simulink model "roach2_fengine_nlb"  (R2013b)
settings: Solver=VariableStepDiscrete  SolverMode=SingleTasking  StartTime=0.0  StopTime=10.0  RelTol=1e-3
undefined symbols (not defined in the file or in its folder): sfp
libraries: xbsIndex_r4 x3316, xps_library x74, casper_library_sources x16, casper_library_misc x7
(part 4 of 38)

== system roach2_fengine_nlb/eq/7 ==
  note: Counter has length nchan=number of channels of the fft.
      | BRAM has length nchan as well. Every input/channel
      | has its own eq value.
      | Top half of the BRAM, has coefficients for first input,
      | second half for the rest.
  note: shared brams have a latency of three
  in : Inport
  sync : Inport  Port=2
  Constant4 : xbsIndex_r4/Constant  const=0  gui_display_data_type=Fixed-point  arith_type=Unsigned  n_bits=18  bin_pt=0  preci_type=Single  exp_width=8  frac_width=24  explicit_period=on  period=1  equ=P=C  opselect=C  inp2=PCIN>>17  opr=+  inp1=P  carry=CIN  dbl_ovrd=off  block_type=constant
  Constant5 : xbsIndex_r4/Constant  const=0  gui_display_data_type=Fixed-point  arith_type=Boolean  n_bits=1  bin_pt=0  preci_type=Single  exp_width=8  frac_width=24  explicit_period=on  period=1  equ=P=C  opselect=C  inp2=PCIN>>17  opr=+  inp1=P  carry=CIN  dbl_ovrd=off  block_type=constant
  Counter : xbsIndex_r4/Counter  cnt_type=Free Running  cnt_to=Inf  operation=Up  start_count=0  cnt_by_val=1  arith_type=Unsigned  n_bits=nchan  bin_pt=0  load_pin=off  rst=on  en=off  explicit_period=off  period=1  dbl_ovrd=off  use_behavioral_HDL=off  implementation=Fabric  use_rpm=on  block_type=counter
      settings: xl_area=[0, 0, 0, 0, 0, 0, 0]
  Delay1 : xbsIndex_r4/Delay  rst=off  infoeditControl=Selection of Reset will increase slice count due to use of real FFs and instead of SRLs  en=off  latency=4  dbl_ovrd=off  reg_retiming=on  block_type=delay
      settings: xl_area=[0, 0, 0, 0, 0, 0, 0]
  Delay11 : xbsIndex_r4/Delay  rst=off  infoeditControl=Selection of Reset will increase slice count due to use of real FFs and instead of SRLs  en=off  latency=4  dbl_ovrd=off  reg_retiming=on  block_type=delay
      settings: xl_area=[0, 0, 0, 0, 0, 0, 0]
  Delay2 : xbsIndex_r4/Delay  rst=off  infoeditControl=Selection of Reset will increase slice count due to use of real FFs and instead of SRLs  en=off  latency=3  dbl_ovrd=off  reg_retiming=off  block_type=delay
      settings: xl_area=[0, 0, 0, 0, 0, 0, 0]
  Delay3 : xbsIndex_r4/Delay  rst=off  infoeditControl=Selection of Reset will increase slice count due to use of real FFs and instead of SRLs  en=off  latency=4  dbl_ovrd=off  reg_retiming=on  block_type=delay
      settings: xl_area=[0, 0, 0, 0, 0, 0, 0]
  Delay4 : xbsIndex_r4/Delay  rst=off  infoeditControl=Selection of Reset will increase slice count due to use of real FFs and instead of SRLs  en=off  latency=5  dbl_ovrd=off  reg_retiming=off  block_type=delay
      settings: xl_area=[0, 0, 0, 0, 0, 0, 0]
  Delay5 : xbsIndex_r4/Delay  rst=off  infoeditControl=Selection of Reset will increase slice count due to use of real FFs and instead of SRLs  en=off  latency=3  dbl_ovrd=off  reg_retiming=off  block_type=delay
      settings: xl_area=[0, 0, 0, 0, 0, 0, 0]
  Slice1 : xbsIndex_r4/Slice  nbits=18  boolean_output=off  mode=Lower Bit Location + Width  bit1=0  base1=MSB of Input  bit0=0  base0=LSB of Input  dbl_ovrd=off  block_type=slice
      settings: block_version=10.1.3
  coeffs : Subsystem  Tag=xps:bram  AncestorBlock=xps_library/Shared BRAM  mask{arith_type=Unsigned, addr_width=nchan, data_width=32, reg_prim_output=on, reg_core_output=on, optimization=Minimum_Area, data_bin_pt=0, init_vals=[0:2^10-1], sample_rate=1}
      mask prompts: arith_type "Output Data Type"; addr_width "Address width"; data_width "Data Width"; reg_prim_output "Register Primitive Output"; reg_core_output "Register Core Output"; data_bin_pt "Data Binary Point"; init_vals "Initial 32-bit values (simulation only)"; sample_rate "Sample rate"
      mask init:
      | shared_bram_mask;
      mask TypeOptions arith_type: Unsigned | Signed  (2's comp)
      mask TypeOptions data_width: 8 | 16 | 32 | 64 | 128
      mask TypeOptions optimization: Minimum_Area | Low_Power
  round : Subsystem
      settings: AttributesFormatString=latency=5
  dout : Outport
  sync_out : Outport  Port=2
  clip : Outport  Port=3
  wires:
  Constant4/1 -> coeffs/2(data_in)
  Constant5/1 -> coeffs/3(we)
  sync/1 -> Counter/1, Delay5/1
  round/1(dout) -> dout/1
  in/1 -> Delay2/1
  Delay4/1 -> sync_out/1
  round/2(clip) -> clip/1
  coeffs/1(data_out) -> Slice1/1
  Counter/1 -> coeffs/1(addr)
  Delay1/1 -> round/2(scale)
  Slice1/1 -> Delay1/1
  Delay11/1 -> round/1(din)
  Delay2/1 -> Delay11/1
  Delay3/1 -> Delay4/1
  Delay5/1 -> Delay3/1

== system roach2_fengine_nlb/eq/8 ==
  note: shared brams have a latency of three
  note: Counter has length nchan=number of channels of the fft.
      | BRAM has length nchan as well. Every input/channel
      | has its own eq value.
      | Top half of the BRAM, has coefficients for first input,
      | second half for the rest.
  in : Inport
  sync : Inport  Port=2
  Constant4 : xbsIndex_r4/Constant  const=0  gui_display_data_type=Fixed-point  arith_type=Unsigned  n_bits=18  bin_pt=0  preci_type=Single  exp_width=8  frac_width=24  explicit_period=on  period=1  equ=P=C  opselect=C  inp2=PCIN>>17  opr=+  inp1=P  carry=CIN  dbl_ovrd=off  block_type=constant
  Constant5 : xbsIndex_r4/Constant  const=0  gui_display_data_type=Fixed-point  arith_type=Boolean  n_bits=1  bin_pt=0  preci_type=Single  exp_width=8  frac_width=24  explicit_period=on  period=1  equ=P=C  opselect=C  inp2=PCIN>>17  opr=+  inp1=P  carry=CIN  dbl_ovrd=off  block_type=constant
  Counter : xbsIndex_r4/Counter  cnt_type=Free Running  cnt_to=Inf  operation=Up  start_count=0  cnt_by_val=1  arith_type=Unsigned  n_bits=nchan  bin_pt=0  load_pin=off  rst=on  en=off  explicit_period=off  period=1  dbl_ovrd=off  use_behavioral_HDL=off  implementation=Fabric  use_rpm=on  block_type=counter
      settings: xl_area=[0, 0, 0, 0, 0, 0, 0]
  Delay1 : xbsIndex_r4/Delay  rst=off  infoeditControl=Selection of Reset will increase slice count due to use of real FFs and instead of SRLs  en=off  latency=4  dbl_ovrd=off  reg_retiming=on  block_type=delay
      settings: xl_area=[0, 0, 0, 0, 0, 0, 0]
  Delay11 : xbsIndex_r4/Delay  rst=off  infoeditControl=Selection of Reset will increase slice count due to use of real FFs and instead of SRLs  en=off  latency=4  dbl_ovrd=off  reg_retiming=on  block_type=delay
      settings: xl_area=[0, 0, 0, 0, 0, 0, 0]
  Delay2 : xbsIndex_r4/Delay  rst=off  infoeditControl=Selection of Reset will increase slice count due to use of real FFs and instead of SRLs  en=off  latency=3  dbl_ovrd=off  reg_retiming=off  block_type=delay
      settings: xl_area=[0, 0, 0, 0, 0, 0, 0]
  Delay3 : xbsIndex_r4/Delay  rst=off  infoeditControl=Selection of Reset will increase slice count due to use of real FFs and instead of SRLs  en=off  latency=4  dbl_ovrd=off  reg_retiming=on  block_type=delay
      settings: xl_area=[0, 0, 0, 0, 0, 0, 0]
  Delay4 : xbsIndex_r4/Delay  rst=off  infoeditControl=Selection of Reset will increase slice count due to use of real FFs and instead of SRLs  en=off  latency=5  dbl_ovrd=off  reg_retiming=off  block_type=delay
      settings: xl_area=[0, 0, 0, 0, 0, 0, 0]
  Delay5 : xbsIndex_r4/Delay  rst=off  infoeditControl=Selection of Reset will increase slice count due to use of real FFs and instead of SRLs  en=off  latency=3  dbl_ovrd=off  reg_retiming=off  block_type=delay
      settings: xl_area=[0, 0, 0, 0, 0, 0, 0]
  Slice1 : xbsIndex_r4/Slice  nbits=18  boolean_output=off  mode=Lower Bit Location + Width  bit1=0  base1=MSB of Input  bit0=0  base0=LSB of Input  dbl_ovrd=off  block_type=slice
      settings: block_version=10.1.3
  coeffs : Subsystem  Tag=xps:bram  AncestorBlock=xps_library/Shared BRAM  mask{arith_type=Unsigned, addr_width=nchan, data_width=32, reg_prim_output=on, reg_core_output=on, optimization=Minimum_Area, data_bin_pt=0, init_vals=[0:2^10-1], sample_rate=1}
      mask prompts: arith_type "Output Data Type"; addr_width "Address width"; data_width "Data Width"; reg_prim_output "Register Primitive Output"; reg_core_output "Register Core Output"; data_bin_pt "Data Binary Point"; init_vals "Initial 32-bit values (simulation only)"; sample_rate "Sample rate"
      mask init:
      | shared_bram_mask;
      mask TypeOptions arith_type: Unsigned | Signed  (2's comp)
      mask TypeOptions data_width: 8 | 16 | 32 | 64 | 128
      mask TypeOptions optimization: Minimum_Area | Low_Power
  round : Subsystem
      settings: AttributesFormatString=latency=5
  dout : Outport
  sync_out : Outport  Port=2
  clip : Outport  Port=3
  wires:
  Delay5/1 -> Delay3/1
  Delay3/1 -> Delay4/1
  Delay2/1 -> Delay11/1
  Delay11/1 -> round/1(din)
  Slice1/1 -> Delay1/1
  Delay1/1 -> round/2(scale)
  Counter/1 -> coeffs/1(addr)
  coeffs/1(data_out) -> Slice1/1
  round/2(clip) -> clip/1
  Delay4/1 -> sync_out/1
  in/1 -> Delay2/1
  round/1(dout) -> dout/1
  sync/1 -> Delay5/1, Counter/1
  Constant5/1 -> coeffs/3(we)
  Constant4/1 -> coeffs/2(data_in)

== system roach2_fengine_nlb/eq/9 ==
  note: shared brams have a latency of three
  note: Counter has length nchan=number of channels of the fft.
      | BRAM has length nchan as well. Every input/channel
      | has its own eq value.
      | Top half of the BRAM, has coefficients for first input,
      | second half for the rest.
  in : Inport
  sync : Inport  Port=2
  Constant4 : xbsIndex_r4/Constant  const=0  gui_display_data_type=Fixed-point  arith_type=Unsigned  n_bits=18  bin_pt=0  preci_type=Single  exp_width=8  frac_width=24  explicit_period=on  period=1  equ=P=C  opselect=C  inp2=PCIN>>17  opr=+  inp1=P  carry=CIN  dbl_ovrd=off  block_type=constant
  Constant5 : xbsIndex_r4/Constant  const=0  gui_display_data_type=Fixed-point  arith_type=Boolean  n_bits=1  bin_pt=0  preci_type=Single  exp_width=8  frac_width=24  explicit_period=on  period=1  equ=P=C  opselect=C  inp2=PCIN>>17  opr=+  inp1=P  carry=CIN  dbl_ovrd=off  block_type=constant
  Counter : xbsIndex_r4/Counter  cnt_type=Free Running  cnt_to=Inf  operation=Up  start_count=0  cnt_by_val=1  arith_type=Unsigned  n_bits=nchan  bin_pt=0  load_pin=off  rst=on  en=off  explicit_period=off  period=1  dbl_ovrd=off  use_behavioral_HDL=off  implementation=Fabric  use_rpm=on  block_type=counter
      settings: xl_area=[0, 0, 0, 0, 0, 0, 0]
  Delay1 : xbsIndex_r4/Delay  rst=off  infoeditControl=Selection of Reset will increase slice count due to use of real FFs and instead of SRLs  en=off  latency=4  dbl_ovrd=off  reg_retiming=on  block_type=delay
      settings: xl_area=[0, 0, 0, 0, 0, 0, 0]
  Delay11 : xbsIndex_r4/Delay  rst=off  infoeditControl=Selection of Reset will increase slice count due to use of real FFs and instead of SRLs  en=off  latency=4  dbl_ovrd=off  reg_retiming=on  block_type=delay
      settings: xl_area=[0, 0, 0, 0, 0, 0, 0]
  Delay2 : xbsIndex_r4/Delay  rst=off  infoeditControl=Selection of Reset will increase slice count due to use of real FFs and instead of SRLs  en=off  latency=3  dbl_ovrd=off  reg_retiming=off  block_type=delay
      settings: xl_area=[0, 0, 0, 0, 0, 0, 0]
  Delay3 : xbsIndex_r4/Delay  rst=off  infoeditControl=Selection of Reset will increase slice count due to use of real FFs and instead of SRLs  en=off  latency=4  dbl_ovrd=off  reg_retiming=on  block_type=delay
      settings: xl_area=[0, 0, 0, 0, 0, 0, 0]
  Delay4 : xbsIndex_r4/Delay  rst=off  infoeditControl=Selection of Reset will increase slice count due to use of real FFs and instead of SRLs  en=off  latency=5  dbl_ovrd=off  reg_retiming=off  block_type=delay
      settings: xl_area=[0, 0, 0, 0, 0, 0, 0]
  Delay5 : xbsIndex_r4/Delay  rst=off  infoeditControl=Selection of Reset will increase slice count due to use of real FFs and instead of SRLs  en=off  latency=3  dbl_ovrd=off  reg_retiming=off  block_type=delay
      settings: xl_area=[0, 0, 0, 0, 0, 0, 0]
  Slice1 : xbsIndex_r4/Slice  nbits=18  boolean_output=off  mode=Lower Bit Location + Width  bit1=0  base1=MSB of Input  bit0=0  base0=LSB of Input  dbl_ovrd=off  block_type=slice
      settings: block_version=10.1.3
  coeffs : Subsystem  Tag=xps:bram  AncestorBlock=xps_library/Shared BRAM  mask{arith_type=Unsigned, addr_width=nchan, data_width=32, reg_prim_output=on, reg_core_output=on, optimization=Minimum_Area, data_bin_pt=0, init_vals=[0:2^10-1], sample_rate=1}
      mask prompts: arith_type "Output Data Type"; addr_width "Address width"; data_width "Data Width"; reg_prim_output "Register Primitive Output"; reg_core_output "Register Core Output"; data_bin_pt "Data Binary Point"; init_vals "Initial 32-bit values (simulation only)"; sample_rate "Sample rate"
      mask init:
      | shared_bram_mask;
      mask TypeOptions arith_type: Unsigned | Signed  (2's comp)
      mask TypeOptions data_width: 8 | 16 | 32 | 64 | 128
      mask TypeOptions optimization: Minimum_Area | Low_Power
  round : Subsystem
      settings: AttributesFormatString=latency=5
  dout : Outport
  sync_out : Outport  Port=2
  clip : Outport  Port=3
  wires:
  Delay5/1 -> Delay3/1
  Delay3/1 -> Delay4/1
  Delay2/1 -> Delay11/1
  Delay11/1 -> round/1(din)
  Slice1/1 -> Delay1/1
  Delay1/1 -> round/2(scale)
  Counter/1 -> coeffs/1(addr)
  coeffs/1(data_out) -> Slice1/1
  round/2(clip) -> clip/1
  Delay4/1 -> sync_out/1
  in/1 -> Delay2/1
  round/1(dout) -> dout/1
  sync/1 -> Delay5/1, Counter/1
  Constant5/1 -> coeffs/3(we)
  Constant4/1 -> coeffs/2(data_in)

== system roach2_fengine_nlb/eq/eq_snap ==
  In1 : Inport
  In2 : Inport  Port=2
  In3 : Inport  Port=3
  In4 : Inport  Port=4
  BitBasher : xbsIndex_r4/BitBasher  bitexpr=|  display_expr=off  sr_1=1  arith_type1=Unsigned  bin_pt1=0  sr_2=2  arith_type2=Unsigned  bin_pt2=0  sr_3=3  arith_type3=Unsigned  bin_pt3=0  sr_4=4  arith_type4=Unsigned  bin_pt4=0  dbl_ovrd=off  block_type=bitbasher
      | <!DOCTYPE HTML PUBLIC "-//W3C//DTD HTML 4.0//EN" "http://www.w3.org/TR/REC-html40/strict.dtd">
      | <html><head><meta name="qrichtext" content="1" /><style type="text/css">
      | p, li { white-space: pre-wrap; }
      | </style></head><body style=" font-family:'Sans'; font-size:10pt; font-weight:400; font-style:normal;">
      | <p style=" margin-top:12px; margin-bottom:12px; margin-left:0px; margin-right:0px; -qt-block-indent:0; text-indent:0px;"><span style=" font-family:'MS Shell Dlg'; font-size:8pt;">w32={d8,c8,b8,a8}</span></p></body></html>
  Delay : xbsIndex_r4/Delay  rst=off  infoeditControl=Selection of Reset will increase slice count due to use of real FFs and instead of SRLs  en=off  latency=3  dbl_ovrd=off  reg_retiming=on  block_type=delay
  tag scope: eq_snap=global
  wires:
  BitBasher/1 -> Delay/1
  Delay/1 -> [eq_snap]
  In1/1 -> BitBasher/1
  In2/1 -> BitBasher/2
  In3/1 -> BitBasher/3
  In4/1 -> BitBasher/4

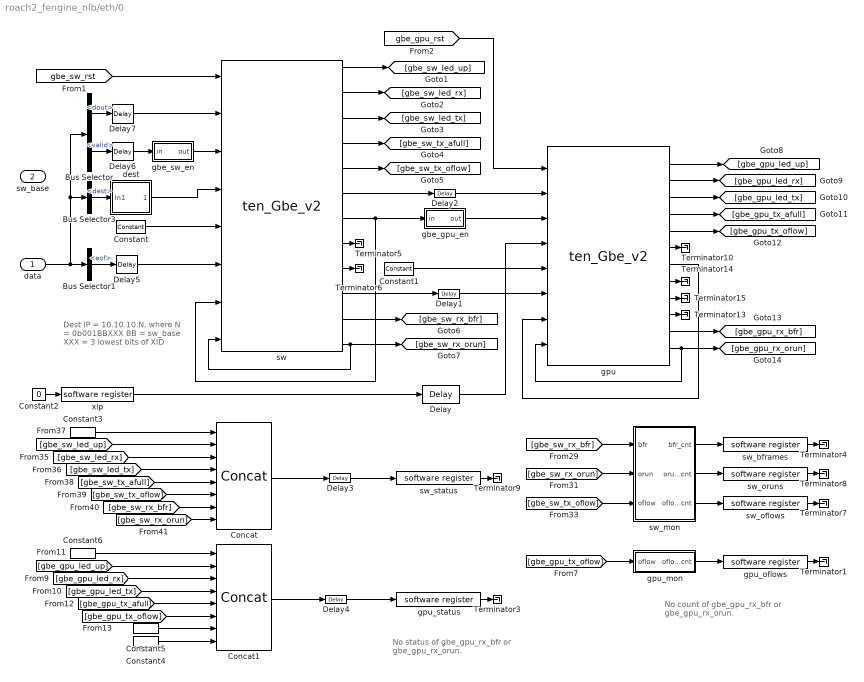
== system roach2_fengine_nlb/eth/0 ==
  note: Dest IP = 10.10.10.N, where
      | N = 0b001BBXXX
      | BB = sw_base
      | XXX = 3 lowest bits of XID
  note: No count of gbe_gpu_rx_bfr or gbe_gpu_rx_orun.
  note: No status of gbe_gpu_rx_bfr or gbe_gpu_rx_orun.
  data : Inport
  sw_base : Inport  Port=2
  Bus Selector : BusSelector  OutputSignals=dout,valid
  Bus Selector1 : BusSelector  OutputSignals=eof
  Bus Selector3 : BusSelector  OutputSignals=dest
  Concat : xbsIndex_r4/Concat  num_inputs=8  dbl_ovrd=off  block_type=concat
  Concat1 : xbsIndex_r4/Concat  num_inputs=8  dbl_ovrd=off  block_type=concat
  Constant : xbsIndex_r4/Constant  const=8511  gui_display_data_type=Fixed-point  arith_type=Unsigned  n_bits=16  bin_pt=0  preci_type=Single  exp_width=8  frac_width=24  explicit_period=on  period=1  equ=P=C  opselect=C  inp2=PCIN>>17  opr=+  inp1=P  carry=CIN  dbl_ovrd=off  block_type=constant
  Constant1 : xbsIndex_r4/Constant  const=8511  gui_display_data_type=Fixed-point  arith_type=Unsigned  n_bits=16  bin_pt=0  preci_type=Single  exp_width=8  frac_width=24  explicit_period=on  period=1  equ=P=C  opselect=C  inp2=PCIN>>17  opr=+  inp1=P  carry=CIN  dbl_ovrd=off  block_type=constant
  Constant2 : Constant  Value=0
  Constant3 : xbsIndex_r4/Constant  const=0  gui_display_data_type=Fixed-point  arith_type=Unsigned  n_bits=25  bin_pt=0  preci_type=Single  exp_width=8  frac_width=24  explicit_period=on  period=1  equ=P=C  opselect=C  inp2=PCIN>>17  opr=+  inp1=P  carry=CIN  dbl_ovrd=off  block_type=constant
      settings: block_version=11.4
  Constant4 : xbsIndex_r4/Constant  const=0  gui_display_data_type=Fixed-point  arith_type=Unsigned  n_bits=1  bin_pt=0  preci_type=Single  exp_width=8  frac_width=24  explicit_period=on  period=1  equ=P=C  opselect=C  inp2=PCIN>>17  opr=+  inp1=P  carry=CIN  dbl_ovrd=off  block_type=constant
      settings: block_version=11.4
  Constant5 : xbsIndex_r4/Constant  const=0  gui_display_data_type=Fixed-point  arith_type=Unsigned  n_bits=1  bin_pt=0  preci_type=Single  exp_width=8  frac_width=24  explicit_period=on  period=1  equ=P=C  opselect=C  inp2=PCIN>>17  opr=+  inp1=P  carry=CIN  dbl_ovrd=off  block_type=constant
      settings: block_version=11.4
  Constant6 : xbsIndex_r4/Constant  const=0  gui_display_data_type=Fixed-point  arith_type=Unsigned  n_bits=25  bin_pt=0  preci_type=Single  exp_width=8  frac_width=24  explicit_period=on  period=1  equ=P=C  opselect=C  inp2=PCIN>>17  opr=+  inp1=P  carry=CIN  dbl_ovrd=off  block_type=constant
      settings: block_version=11.4
  Delay{,1..4} (5 alike) : xbsIndex_r4/Delay  rst=off  infoeditControl=Selection of Reset will increase slice count due to use of real FFs and instead of SRLs  en=off  latency=1  dbl_ovrd=off  reg_retiming=off  block_type=delay
  Delay5 : xbsIndex_r4/Delay  rst=off  infoeditControl=Selection of Reset will increase slice count due to use of real FFs and instead of SRLs  en=off  latency=3  dbl_ovrd=off  reg_retiming=off  block_type=delay
  Delay6 : xbsIndex_r4/Delay  rst=off  infoeditControl=Selection of Reset will increase slice count due to use of real FFs and instead of SRLs  en=off  latency=3  dbl_ovrd=off  reg_retiming=off  block_type=delay
  Delay7 : xbsIndex_r4/Delay  rst=off  infoeditControl=Selection of Reset will increase slice count due to use of real FFs and instead of SRLs  en=off  latency=3  dbl_ovrd=off  reg_retiming=off  block_type=delay
  Terminator{1,3..10,13..15} (12 alike) : Terminator
  dest : Subsystem
  gbe_gpu_en : Subsystem
  gbe_sw_en : Subsystem
  gpu : xps_library/ten_Gbe_v2  Tag=xps:tengbe_v2  flavour=sfp+  slot=0  port_r1=0  port_r2_cx4=0  port_r2_sfpp=1  rx_dist_ram=on  large_frames=on  show_param=on  pre_emph_r2=0.74  pre_emph=3  post_emph_r2=0.18  rxeqmix_r2=7  swing_r2=940  swing=800  fab_en=on  fab_mac=hex2dec('0202c0a80201')  fab_ip=hex2dec('c0a80201')  fab_udp=8511  fab_gate=1  cpu_rx_en=off  cpu_tx_en=off
  gpu_mon : Subsystem
  gpu_oflows : xps_library/software register  Tag=xps:sw_reg  io_dir=To Processor  arith_type=Unsigned  bitwidth=32  bin_pt=0  sample_period=1  gw_name=roach2_fengine_orig_eth_0_gpu_oflows_user_data_in
  gpu_status : xps_library/software register  Tag=xps:sw_reg  io_dir=To Processor  arith_type=Unsigned  bitwidth=32  bin_pt=0  sample_period=1  gw_name=roach2_fengine_orig_eth_0_gpu_status_user_data_in
  sw : xps_library/ten_Gbe_v2  Tag=xps:tengbe_v2  flavour=sfp+  slot=0  port_r1=0  port_r2_cx4=0  port_r2_sfpp=0  rx_dist_ram=off  large_frames=on  show_param=on  pre_emph_r2=0.74  pre_emph=3  post_emph_r2=0.18  rxeqmix_r2=7  swing_r2=940  swing=800  fab_en=on  fab_mac=hex2dec('02020a0a0a20')  fab_ip=hex2dec('0a0a0a20')  fab_udp=8511  fab_gate=1  cpu_rx_en=off  cpu_tx_en=off
  sw_bframes : xps_library/software register  Tag=xps:sw_reg  io_dir=To Processor  arith_type=Unsigned  bitwidth=32  bin_pt=0  sample_period=1  gw_name=roach2_fengine_orig_eth_0_sw_bframes_user_data_in
  sw_mon : Subsystem
  sw_oflows : xps_library/software register  Tag=xps:sw_reg  io_dir=To Processor  arith_type=Unsigned  bitwidth=32  bin_pt=0  sample_period=1  gw_name=roach2_fengine_orig_eth_0_sw_oflows_user_data_in
  sw_oruns : xps_library/software register  Tag=xps:sw_reg  io_dir=To Processor  arith_type=Unsigned  bitwidth=32  bin_pt=0  sample_period=1  gw_name=roach2_fengine_orig_eth_0_sw_oruns_user_data_in
  sw_status : xps_library/software register  Tag=xps:sw_reg  io_dir=To Processor  arith_type=Unsigned  bitwidth=32  bin_pt=0  sample_period=1  gw_name=roach2_fengine_orig_eth_0_sw_status_user_data_in
  xip : xps_library/software register  Tag=xps:sw_reg  io_dir=From Processor  arith_type=Unsigned  bitwidth=32  bin_pt=0  sample_period=1  gw_name=roach2_fengine_orig_eth_0_xip_user_data_out
  wires:
  sw_status/1 -> Terminator9/1
  sw_oruns/1 -> Terminator8/1
  sw_oflows/1 -> Terminator7/1
  sw_bframes/1 -> Terminator4/1
  gpu_status/1 -> Terminator3/1
  gpu_oflows/1 -> Terminator1/1
  Bus Selector/1 -> Delay7/1  "<dout>"
  Bus Selector/2 -> Delay6/1  "<valid>"
  data/1 -> Bus Selector3/1, Bus Selector/1, Bus Selector1/1
  Bus Selector1/1 -> Delay5/1  "<eof>"
  Constant/1 -> sw/5
  sw/6 -> Delay2/1
  sw/7 -> sw/7, gbe_gpu_en/1(in)
  sw/10 -> Delay1/1
  dest/1(Out1) -> sw/4
  Constant1/1 -> gpu/5
  sw/12 -> sw/8, [gbe_sw_rx_orun]
  gpu/12 -> gpu/8, [gbe_gpu_rx_orun]
  gpu/7 -> gpu/7
  [gbe_sw_rst] -> sw/1
  [gbe_gpu_rst] -> gpu/1
  gbe_sw_en/1(out) -> sw/3
  gbe_gpu_en/1(out) -> gpu/3
  sw/1 -> [gbe_sw_led_up]
  sw/2 -> [gbe_sw_led_rx]
  sw/3 -> [gbe_sw_led_tx]
  sw/4 -> [gbe_sw_tx_afull]
  sw/5 -> [gbe_sw_tx_oflow]
  sw/8 -> Terminator5/1
  sw/9 -> Terminator6/1
  sw/11 -> [gbe_sw_rx_bfr]
  gpu/1 -> [gbe_gpu_led_up]
  gpu/2 -> [gbe_gpu_led_rx]
  gpu/3 -> [gbe_gpu_led_tx]
  gpu/4 -> [gbe_gpu_tx_afull]
  gpu/5 -> [gbe_gpu_tx_oflow]
  gpu/6 -> Terminator10/1
  gpu/8 -> Terminator14/1
  gpu/9 -> Terminator15/1
  gpu/10 -> Terminator13/1
  gpu/11 -> [gbe_gpu_rx_bfr]
  [gbe_sw_rx_bfr] -> sw_mon/1(bfr)
  [gbe_sw_rx_orun] -> sw_mon/2(orun)
  [gbe_sw_tx_oflow] -> sw_mon/3(oflow)
  Concat/1 -> Delay3/1
  Constant3/1 -> Concat/1
  [gbe_sw_led_up] -> Concat/2
  [gbe_sw_led_rx] -> Concat/3
  [gbe_sw_led_tx] -> Concat/4
  [gbe_sw_tx_afull] -> Concat/5
  [gbe_sw_tx_oflow] -> Concat/6
  [gbe_sw_rx_bfr] -> Concat/7
  [gbe_sw_rx_orun] -> Concat/8
  Concat1/1 -> Delay4/1
  Constant6/1 -> Concat1/1
  [gbe_gpu_led_up] -> Concat1/2
  [gbe_gpu_led_rx] -> Concat1/3
  [gbe_gpu_led_tx] -> Concat1/4
  [gbe_gpu_tx_afull] -> Concat1/5
  [gbe_gpu_tx_oflow] -> Concat1/6
  Constant5/1 -> Concat1/7
  Constant4/1 -> Concat1/8
  Bus Selector3/1 -> dest/1(In1)  "<dest>"
  Delay/1 -> gpu/4
  xip/1 -> Delay/1
  Constant2/1 -> xip/1
  Delay2/1 -> gpu/2
  Delay1/1 -> gpu/6
  Delay3/1 -> sw_status/1
  Delay4/1 -> gpu_status/1
  sw_mon/1(bfr_cnt) -> sw_bframes/1
  sw_mon/3(oflow_cnt) -> sw_oflows/1
  sw_mon/2(orun_cnt) -> sw_oruns/1
  gpu_mon/1(oflow_cnt) -> gpu_oflows/1
  [gbe_gpu_tx_oflow] -> gpu_mon/1(oflow)
  Delay5/1 -> sw/6
  Delay6/1 -> gbe_sw_en/1(in)
  Delay7/1 -> sw/2

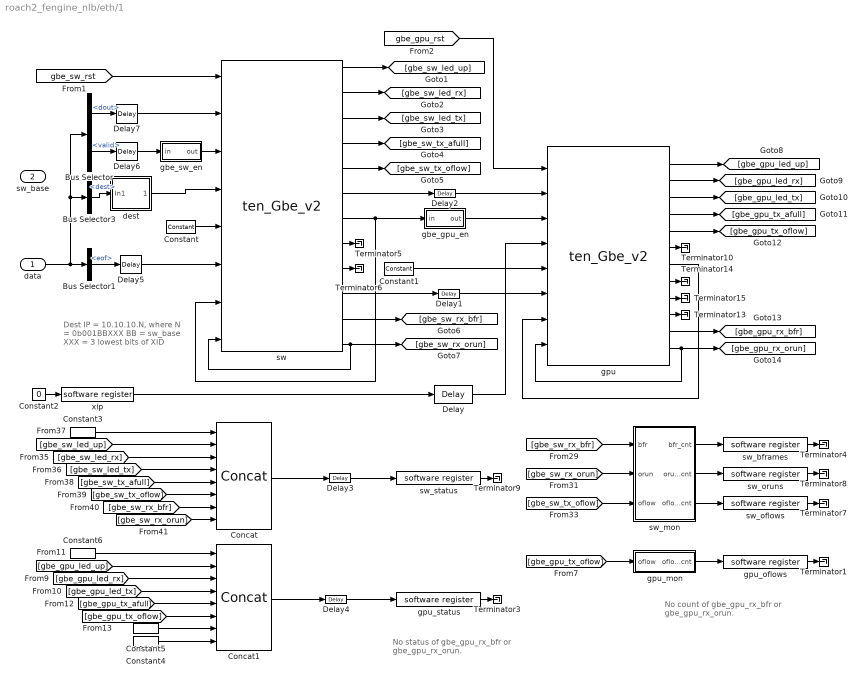
== system roach2_fengine_nlb/eth/1 ==
  note: No status of gbe_gpu_rx_bfr or gbe_gpu_rx_orun.
  note: No count of gbe_gpu_rx_bfr or gbe_gpu_rx_orun.
  note: Dest IP = 10.10.10.N, where
      | N = 0b001BBXXX
      | BB = sw_base
      | XXX = 3 lowest bits of XID
  data : Inport
  sw_base : Inport  Port=2
  Bus Selector : BusSelector  OutputSignals=dout,valid
  Bus Selector1 : BusSelector  OutputSignals=eof
  Bus Selector3 : BusSelector  OutputSignals=dest
  Concat : xbsIndex_r4/Concat  num_inputs=8  dbl_ovrd=off  block_type=concat
  Concat1 : xbsIndex_r4/Concat  num_inputs=8  dbl_ovrd=off  block_type=concat
  Constant : xbsIndex_r4/Constant  const=8511  gui_display_data_type=Fixed-point  arith_type=Unsigned  n_bits=16  bin_pt=0  preci_type=Single  exp_width=8  frac_width=24  explicit_period=on  period=1  equ=P=C  opselect=C  inp2=PCIN>>17  opr=+  inp1=P  carry=CIN  dbl_ovrd=off  block_type=constant
  Constant1 : xbsIndex_r4/Constant  const=8511  gui_display_data_type=Fixed-point  arith_type=Unsigned  n_bits=16  bin_pt=0  preci_type=Single  exp_width=8  frac_width=24  explicit_period=on  period=1  equ=P=C  opselect=C  inp2=PCIN>>17  opr=+  inp1=P  carry=CIN  dbl_ovrd=off  block_type=constant
  Constant2 : Constant  Value=0
  Constant3 : xbsIndex_r4/Constant  const=0  gui_display_data_type=Fixed-point  arith_type=Unsigned  n_bits=25  bin_pt=0  preci_type=Single  exp_width=8  frac_width=24  explicit_period=on  period=1  equ=P=C  opselect=C  inp2=PCIN>>17  opr=+  inp1=P  carry=CIN  dbl_ovrd=off  block_type=constant
      settings: block_version=11.4
  Constant4 : xbsIndex_r4/Constant  const=0  gui_display_data_type=Fixed-point  arith_type=Unsigned  n_bits=1  bin_pt=0  preci_type=Single  exp_width=8  frac_width=24  explicit_period=on  period=1  equ=P=C  opselect=C  inp2=PCIN>>17  opr=+  inp1=P  carry=CIN  dbl_ovrd=off  block_type=constant
      settings: block_version=11.4
  Constant5 : xbsIndex_r4/Constant  const=0  gui_display_data_type=Fixed-point  arith_type=Unsigned  n_bits=1  bin_pt=0  preci_type=Single  exp_width=8  frac_width=24  explicit_period=on  period=1  equ=P=C  opselect=C  inp2=PCIN>>17  opr=+  inp1=P  carry=CIN  dbl_ovrd=off  block_type=constant
      settings: block_version=11.4
  Constant6 : xbsIndex_r4/Constant  const=0  gui_display_data_type=Fixed-point  arith_type=Unsigned  n_bits=25  bin_pt=0  preci_type=Single  exp_width=8  frac_width=24  explicit_period=on  period=1  equ=P=C  opselect=C  inp2=PCIN>>17  opr=+  inp1=P  carry=CIN  dbl_ovrd=off  block_type=constant
      settings: block_version=11.4
  Delay{,1..4} (5 alike) : xbsIndex_r4/Delay  rst=off  infoeditControl=Selection of Reset will increase slice count due to use of real FFs and instead of SRLs  en=off  latency=1  dbl_ovrd=off  reg_retiming=off  block_type=delay
  Delay5 : xbsIndex_r4/Delay  rst=off  infoeditControl=Selection of Reset will increase slice count due to use of real FFs and instead of SRLs  en=off  latency=3  dbl_ovrd=off  reg_retiming=off  block_type=delay
  Delay6 : xbsIndex_r4/Delay  rst=off  infoeditControl=Selection of Reset will increase slice count due to use of real FFs and instead of SRLs  en=off  latency=3  dbl_ovrd=off  reg_retiming=off  block_type=delay
  Delay7 : xbsIndex_r4/Delay  rst=off  infoeditControl=Selection of Reset will increase slice count due to use of real FFs and instead of SRLs  en=off  latency=3  dbl_ovrd=off  reg_retiming=off  block_type=delay
  Terminator{1,3..10,13..15} (12 alike) : Terminator
  dest : Subsystem
  gbe_gpu_en : Subsystem
  gbe_sw_en : Subsystem
  gpu : xps_library/ten_Gbe_v2  Tag=xps:tengbe_v2  flavour=sfp+  slot=0  port_r1=0  port_r2_cx4=0  port_r2_sfpp=3  rx_dist_ram=on  large_frames=on  show_param=on  pre_emph_r2=0.74  pre_emph=3  post_emph_r2=0.18  rxeqmix_r2=7  swing_r2=940  swing=800  fab_en=on  fab_mac=hex2dec('0202c0a80301')  fab_ip=hex2dec('c0a80301')  fab_udp=8511  fab_gate=1  cpu_rx_en=off  cpu_tx_en=off
  gpu_mon : Subsystem
  gpu_oflows : xps_library/software register  Tag=xps:sw_reg  io_dir=To Processor  arith_type=Unsigned  bitwidth=32  bin_pt=0  sample_period=1  gw_name=roach2_fengine_orig_eth_1_gpu_oflows_user_data_in
  gpu_status : xps_library/software register  Tag=xps:sw_reg  io_dir=To Processor  arith_type=Unsigned  bitwidth=32  bin_pt=0  sample_period=1  gw_name=roach2_fengine_orig_eth_1_gpu_status_user_data_in
  sw : xps_library/ten_Gbe_v2  Tag=xps:tengbe_v2  flavour=sfp+  slot=0  port_r1=0  port_r2_cx4=0  port_r2_sfpp=2  rx_dist_ram=off  large_frames=on  show_param=on  pre_emph_r2=0.74  pre_emph=3  post_emph_r2=0.18  rxeqmix_r2=7  swing_r2=940  swing=800  fab_en=on  fab_mac=hex2dec('02020a0a0a28')  fab_ip=hex2dec('0a0a0a28')  fab_udp=8511  fab_gate=1  cpu_rx_en=off  cpu_tx_en=off
  sw_bframes : xps_library/software register  Tag=xps:sw_reg  io_dir=To Processor  arith_type=Unsigned  bitwidth=32  bin_pt=0  sample_period=1  gw_name=roach2_fengine_orig_eth_1_sw_bframes_user_data_in
  sw_mon : Subsystem
  sw_oflows : xps_library/software register  Tag=xps:sw_reg  io_dir=To Processor  arith_type=Unsigned  bitwidth=32  bin_pt=0  sample_period=1  gw_name=roach2_fengine_orig_eth_1_sw_oflows_user_data_in
  sw_oruns : xps_library/software register  Tag=xps:sw_reg  io_dir=To Processor  arith_type=Unsigned  bitwidth=32  bin_pt=0  sample_period=1  gw_name=roach2_fengine_orig_eth_1_sw_oruns_user_data_in
  sw_status : xps_library/software register  Tag=xps:sw_reg  io_dir=To Processor  arith_type=Unsigned  bitwidth=32  bin_pt=0  sample_period=1  gw_name=roach2_fengine_orig_eth_1_sw_status_user_data_in
  xip : xps_library/software register  Tag=xps:sw_reg  io_dir=From Processor  arith_type=Unsigned  bitwidth=32  bin_pt=0  sample_period=1  gw_name=roach2_fengine_orig_eth_1_xip_user_data_out
  wires:
  [gbe_gpu_tx_oflow] -> gpu_mon/1(oflow)
  gpu_mon/1(oflow_cnt) -> gpu_oflows/1
  sw_mon/2(orun_cnt) -> sw_oruns/1
  sw_mon/3(oflow_cnt) -> sw_oflows/1
  sw_mon/1(bfr_cnt) -> sw_bframes/1
  Delay4/1 -> gpu_status/1
  Delay3/1 -> sw_status/1
  Delay1/1 -> gpu/6
  Delay2/1 -> gpu/2
  Constant2/1 -> xip/1
  xip/1 -> Delay/1
  Delay/1 -> gpu/4
  Bus Selector3/1 -> dest/1(In1)  "<dest>"
  Constant4/1 -> Concat1/8
  Constant5/1 -> Concat1/7
  [gbe_gpu_tx_oflow] -> Concat1/6
  [gbe_gpu_tx_afull] -> Concat1/5
  [gbe_gpu_led_tx] -> Concat1/4
  [gbe_gpu_led_rx] -> Concat1/3
  [gbe_gpu_led_up] -> Concat1/2
  Constant6/1 -> Concat1/1
  Concat1/1 -> Delay4/1
  [gbe_sw_rx_orun] -> Concat/8
  [gbe_sw_rx_bfr] -> Concat/7
  [gbe_sw_tx_oflow] -> Concat/6
  [gbe_sw_tx_afull] -> Concat/5
  [gbe_sw_led_tx] -> Concat/4
  [gbe_sw_led_rx] -> Concat/3
  [gbe_sw_led_up] -> Concat/2
  Constant3/1 -> Concat/1
  Concat/1 -> Delay3/1
  [gbe_sw_tx_oflow] -> sw_mon/3(oflow)
  [gbe_sw_rx_orun] -> sw_mon/2(orun)
  [gbe_sw_rx_bfr] -> sw_mon/1(bfr)
  gpu/11 -> [gbe_gpu_rx_bfr]
  gpu/10 -> Terminator13/1
  gpu/9 -> Terminator15/1
  gpu/8 -> Terminator14/1
  gpu/6 -> Terminator10/1
  gpu/5 -> [gbe_gpu_tx_oflow]
  gpu/4 -> [gbe_gpu_tx_afull]
  gpu/3 -> [gbe_gpu_led_tx]
  gpu/2 -> [gbe_gpu_led_rx]
  gpu/1 -> [gbe_gpu_led_up]
  sw/11 -> [gbe_sw_rx_bfr]
  sw/9 -> Terminator6/1
  sw/8 -> Terminator5/1
  sw/5 -> [gbe_sw_tx_oflow]
  sw/4 -> [gbe_sw_tx_afull]
  sw/3 -> [gbe_sw_led_tx]
  sw/2 -> [gbe_sw_led_rx]
  sw/1 -> [gbe_sw_led_up]
  gbe_gpu_en/1(out) -> gpu/3
  gbe_sw_en/1(out) -> sw/3
  [gbe_gpu_rst] -> gpu/1
  [gbe_sw_rst] -> sw/1
  gpu/7 -> gpu/7
  gpu/12 -> [gbe_gpu_rx_orun], gpu/8
  sw/12 -> [gbe_sw_rx_orun], sw/8
  Constant1/1 -> gpu/5
  dest/1(Out1) -> sw/4
  sw/10 -> Delay1/1
  sw/7 -> gbe_gpu_en/1(in), sw/7
  sw/6 -> Delay2/1
  Constant/1 -> sw/5
  Bus Selector1/1 -> Delay5/1  "<eof>"
  data/1 -> Bus Selector1/1, Bus Selector/1, Bus Selector3/1
  Bus Selector/2 -> Delay6/1  "<valid>"
  Bus Selector/1 -> Delay7/1  "<dout>"
  gpu_oflows/1 -> Terminator1/1
  gpu_status/1 -> Terminator3/1
  sw_bframes/1 -> Terminator4/1
  sw_oflows/1 -> Terminator7/1
  sw_oruns/1 -> Terminator8/1
  sw_status/1 -> Terminator9/1
  Delay6/1 -> gbe_sw_en/1(in)
  Delay7/1 -> sw/2
  Delay5/1 -> sw/6

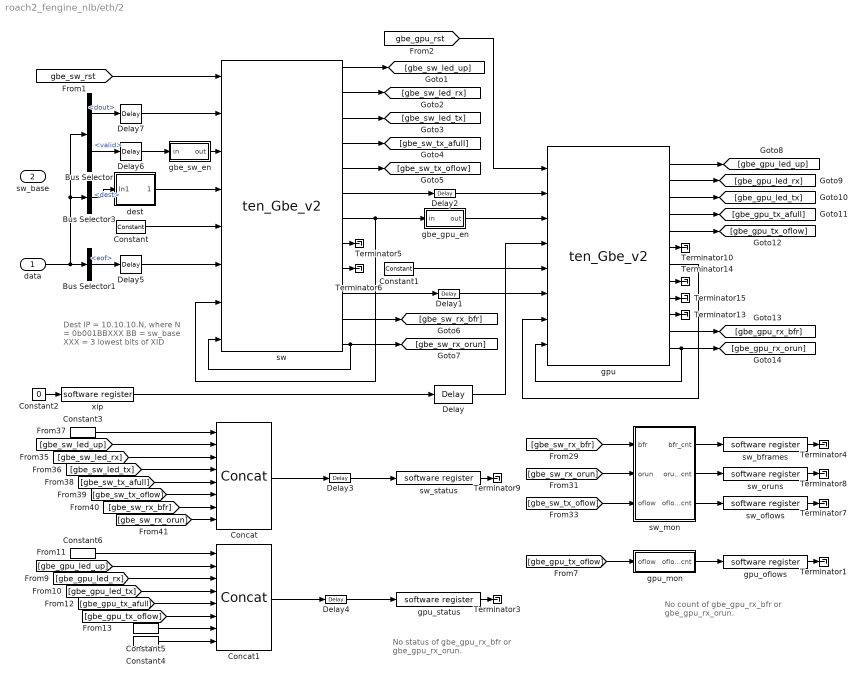
== system roach2_fengine_nlb/eth/2 ==
  note: No status of gbe_gpu_rx_bfr or gbe_gpu_rx_orun.
  note: No count of gbe_gpu_rx_bfr or gbe_gpu_rx_orun.
  note: Dest IP = 10.10.10.N, where
      | N = 0b001BBXXX
      | BB = sw_base
      | XXX = 3 lowest bits of XID
  data : Inport
  sw_base : Inport  Port=2
  Bus Selector : BusSelector  OutputSignals=dout,valid
  Bus Selector1 : BusSelector  OutputSignals=eof
  Bus Selector3 : BusSelector  OutputSignals=dest
  Concat : xbsIndex_r4/Concat  num_inputs=8  dbl_ovrd=off  block_type=concat
  Concat1 : xbsIndex_r4/Concat  num_inputs=8  dbl_ovrd=off  block_type=concat
  Constant : xbsIndex_r4/Constant  const=8511  gui_display_data_type=Fixed-point  arith_type=Unsigned  n_bits=16  bin_pt=0  preci_type=Single  exp_width=8  frac_width=24  explicit_period=on  period=1  equ=P=C  opselect=C  inp2=PCIN>>17  opr=+  inp1=P  carry=CIN  dbl_ovrd=off  block_type=constant
  Constant1 : xbsIndex_r4/Constant  const=8511  gui_display_data_type=Fixed-point  arith_type=Unsigned  n_bits=16  bin_pt=0  preci_type=Single  exp_width=8  frac_width=24  explicit_period=on  period=1  equ=P=C  opselect=C  inp2=PCIN>>17  opr=+  inp1=P  carry=CIN  dbl_ovrd=off  block_type=constant
  Constant2 : Constant  Value=0
  Constant3 : xbsIndex_r4/Constant  const=0  gui_display_data_type=Fixed-point  arith_type=Unsigned  n_bits=25  bin_pt=0  preci_type=Single  exp_width=8  frac_width=24  explicit_period=on  period=1  equ=P=C  opselect=C  inp2=PCIN>>17  opr=+  inp1=P  carry=CIN  dbl_ovrd=off  block_type=constant
      settings: block_version=11.4
  Constant4 : xbsIndex_r4/Constant  const=0  gui_display_data_type=Fixed-point  arith_type=Unsigned  n_bits=1  bin_pt=0  preci_type=Single  exp_width=8  frac_width=24  explicit_period=on  period=1  equ=P=C  opselect=C  inp2=PCIN>>17  opr=+  inp1=P  carry=CIN  dbl_ovrd=off  block_type=constant
      settings: block_version=11.4
  Constant5 : xbsIndex_r4/Constant  const=0  gui_display_data_type=Fixed-point  arith_type=Unsigned  n_bits=1  bin_pt=0  preci_type=Single  exp_width=8  frac_width=24  explicit_period=on  period=1  equ=P=C  opselect=C  inp2=PCIN>>17  opr=+  inp1=P  carry=CIN  dbl_ovrd=off  block_type=constant
      settings: block_version=11.4
  Constant6 : xbsIndex_r4/Constant  const=0  gui_display_data_type=Fixed-point  arith_type=Unsigned  n_bits=25  bin_pt=0  preci_type=Single  exp_width=8  frac_width=24  explicit_period=on  period=1  equ=P=C  opselect=C  inp2=PCIN>>17  opr=+  inp1=P  carry=CIN  dbl_ovrd=off  block_type=constant
      settings: block_version=11.4
  Delay{,1..4} (5 alike) : xbsIndex_r4/Delay  rst=off  infoeditControl=Selection of Reset will increase slice count due to use of real FFs and instead of SRLs  en=off  latency=1  dbl_ovrd=off  reg_retiming=off  block_type=delay
  Delay5 : xbsIndex_r4/Delay  rst=off  infoeditControl=Selection of Reset will increase slice count due to use of real FFs and instead of SRLs  en=off  latency=3  dbl_ovrd=off  reg_retiming=off  block_type=delay
  Delay6 : xbsIndex_r4/Delay  rst=off  infoeditControl=Selection of Reset will increase slice count due to use of real FFs and instead of SRLs  en=off  latency=3  dbl_ovrd=off  reg_retiming=off  block_type=delay
  Delay7 : xbsIndex_r4/Delay  rst=off  infoeditControl=Selection of Reset will increase slice count due to use of real FFs and instead of SRLs  en=off  latency=3  dbl_ovrd=off  reg_retiming=off  block_type=delay
  Terminator{1,3..10,13..15} (12 alike) : Terminator
  dest : Subsystem
  gbe_gpu_en : Subsystem
  gbe_sw_en : Subsystem
  gpu : xps_library/ten_Gbe_v2  Tag=xps:tengbe_v2  flavour=sfp+  slot=1  port_r1=0  port_r2_cx4=0  port_r2_sfpp=1  rx_dist_ram=on  large_frames=on  show_param=on  pre_emph_r2=0.74  pre_emph=3  post_emph_r2=0.18  rxeqmix_r2=7  swing_r2=940  swing=800  fab_en=on  fab_mac=hex2dec('0202c0a80401')  fab_ip=hex2dec('c0a80401')  fab_udp=8511  fab_gate=1  cpu_rx_en=off  cpu_tx_en=off
  gpu_mon : Subsystem
  gpu_oflows : xps_library/software register  Tag=xps:sw_reg  io_dir=To Processor  arith_type=Unsigned  bitwidth=32  bin_pt=0  sample_period=1  gw_name=roach2_fengine_orig_eth_2_gpu_oflows_user_data_in
  gpu_status : xps_library/software register  Tag=xps:sw_reg  io_dir=To Processor  arith_type=Unsigned  bitwidth=32  bin_pt=0  sample_period=1  gw_name=roach2_fengine_orig_eth_2_gpu_status_user_data_in
  sw : xps_library/ten_Gbe_v2  Tag=xps:tengbe_v2  flavour=sfp+  slot=1  port_r1=0  port_r2_cx4=0  port_r2_sfpp=0  rx_dist_ram=off  large_frames=on  show_param=on  pre_emph_r2=0.74  pre_emph=3  post_emph_r2=0.18  rxeqmix_r2=7  swing_r2=940  swing=800  fab_en=on  fab_mac=hex2dec('02020a0a0a30')  fab_ip=hex2dec('0a0a0a30')  fab_udp=8511  fab_gate=1  cpu_rx_en=off  cpu_tx_en=off
  sw_bframes : xps_library/software register  Tag=xps:sw_reg  io_dir=To Processor  arith_type=Unsigned  bitwidth=32  bin_pt=0  sample_period=1  gw_name=roach2_fengine_orig_eth_2_sw_bframes_user_data_in
  sw_mon : Subsystem
  sw_oflows : xps_library/software register  Tag=xps:sw_reg  io_dir=To Processor  arith_type=Unsigned  bitwidth=32  bin_pt=0  sample_period=1  gw_name=roach2_fengine_orig_eth_2_sw_oflows_user_data_in
  sw_oruns : xps_library/software register  Tag=xps:sw_reg  io_dir=To Processor  arith_type=Unsigned  bitwidth=32  bin_pt=0  sample_period=1  gw_name=roach2_fengine_orig_eth_2_sw_oruns_user_data_in
  sw_status : xps_library/software register  Tag=xps:sw_reg  io_dir=To Processor  arith_type=Unsigned  bitwidth=32  bin_pt=0  sample_period=1  gw_name=roach2_fengine_orig_eth_2_sw_status_user_data_in
  xip : xps_library/software register  Tag=xps:sw_reg  io_dir=From Processor  arith_type=Unsigned  bitwidth=32  bin_pt=0  sample_period=1  gw_name=roach2_fengine_orig_eth_2_xip_user_data_out
  wires:
  [gbe_gpu_tx_oflow] -> gpu_mon/1(oflow)
  gpu_mon/1(oflow_cnt) -> gpu_oflows/1
  sw_mon/2(orun_cnt) -> sw_oruns/1
  sw_mon/3(oflow_cnt) -> sw_oflows/1
  sw_mon/1(bfr_cnt) -> sw_bframes/1
  Delay4/1 -> gpu_status/1
  Delay3/1 -> sw_status/1
  Delay1/1 -> gpu/6
  Delay2/1 -> gpu/2
  Constant2/1 -> xip/1
  xip/1 -> Delay/1
  Delay/1 -> gpu/4
  Bus Selector3/1 -> dest/1(In1)  "<dest>"
  Constant4/1 -> Concat1/8
  Constant5/1 -> Concat1/7
  [gbe_gpu_tx_oflow] -> Concat1/6
  [gbe_gpu_tx_afull] -> Concat1/5
  [gbe_gpu_led_tx] -> Concat1/4
  [gbe_gpu_led_rx] -> Concat1/3
  [gbe_gpu_led_up] -> Concat1/2
  Constant6/1 -> Concat1/1
  Concat1/1 -> Delay4/1
  [gbe_sw_rx_orun] -> Concat/8
  [gbe_sw_rx_bfr] -> Concat/7
  [gbe_sw_tx_oflow] -> Concat/6
  [gbe_sw_tx_afull] -> Concat/5
  [gbe_sw_led_tx] -> Concat/4
  [gbe_sw_led_rx] -> Concat/3
  [gbe_sw_led_up] -> Concat/2
  Constant3/1 -> Concat/1
  Concat/1 -> Delay3/1
  [gbe_sw_tx_oflow] -> sw_mon/3(oflow)
  [gbe_sw_rx_orun] -> sw_mon/2(orun)
  [gbe_sw_rx_bfr] -> sw_mon/1(bfr)
  gpu/11 -> [gbe_gpu_rx_bfr]
  gpu/10 -> Terminator13/1
  gpu/9 -> Terminator15/1
  gpu/8 -> Terminator14/1
  gpu/6 -> Terminator10/1
  gpu/5 -> [gbe_gpu_tx_oflow]
  gpu/4 -> [gbe_gpu_tx_afull]
  gpu/3 -> [gbe_gpu_led_tx]
  gpu/2 -> [gbe_gpu_led_rx]
  gpu/1 -> [gbe_gpu_led_up]
  sw/11 -> [gbe_sw_rx_bfr]
  sw/9 -> Terminator6/1
  sw/8 -> Terminator5/1
  sw/5 -> [gbe_sw_tx_oflow]
  sw/4 -> [gbe_sw_tx_afull]
  sw/3 -> [gbe_sw_led_tx]
  sw/2 -> [gbe_sw_led_rx]
  sw/1 -> [gbe_sw_led_up]
  gbe_gpu_en/1(out) -> gpu/3
  gbe_sw_en/1(out) -> sw/3
  [gbe_gpu_rst] -> gpu/1
  [gbe_sw_rst] -> sw/1
  gpu/7 -> gpu/7
  gpu/12 -> [gbe_gpu_rx_orun], gpu/8
  sw/12 -> [gbe_sw_rx_orun], sw/8
  Constant1/1 -> gpu/5
  dest/1(Out1) -> sw/4
  sw/10 -> Delay1/1
  sw/7 -> gbe_gpu_en/1(in), sw/7
  sw/6 -> Delay2/1
  Constant/1 -> sw/5
  Bus Selector1/1 -> Delay5/1  "<eof>"
  data/1 -> Bus Selector1/1, Bus Selector/1, Bus Selector3/1
  Bus Selector/2 -> Delay6/1  "<valid>"
  Bus Selector/1 -> Delay7/1  "<dout>"
  gpu_oflows/1 -> Terminator1/1
  gpu_status/1 -> Terminator3/1
  sw_bframes/1 -> Terminator4/1
  sw_oflows/1 -> Terminator7/1
  sw_oruns/1 -> Terminator8/1
  sw_status/1 -> Terminator9/1
  Delay7/1 -> sw/2
  Delay6/1 -> gbe_sw_en/1(in)
  Delay5/1 -> sw/6

== system roach2_fengine_nlb/eth/3 ==
  note: Dest IP = 10.10.10.N, where
      | N = 0b001BBXXX
      | BB = sw_base
      | XXX = 3 lowest bits of XID
  note: No count of gbe_gpu_rx_bfr or gbe_gpu_rx_orun.
  note: No status of gbe_gpu_rx_bfr or gbe_gpu_rx_orun.
  data : Inport
  sw_base : Inport  Port=2
  Bus Selector : BusSelector  OutputSignals=dout,valid
  Bus Selector1 : BusSelector  OutputSignals=eof
  Bus Selector3 : BusSelector  OutputSignals=dest
  Concat : xbsIndex_r4/Concat  num_inputs=8  dbl_ovrd=off  block_type=concat
  Concat1 : xbsIndex_r4/Concat  num_inputs=8  dbl_ovrd=off  block_type=concat
  Constant : xbsIndex_r4/Constant  const=8511  gui_display_data_type=Fixed-point  arith_type=Unsigned  n_bits=16  bin_pt=0  preci_type=Single  exp_width=8  frac_width=24  explicit_period=on  period=1  equ=P=C  opselect=C  inp2=PCIN>>17  opr=+  inp1=P  carry=CIN  dbl_ovrd=off  block_type=constant
  Constant1 : xbsIndex_r4/Constant  const=8511  gui_display_data_type=Fixed-point  arith_type=Unsigned  n_bits=16  bin_pt=0  preci_type=Single  exp_width=8  frac_width=24  explicit_period=on  period=1  equ=P=C  opselect=C  inp2=PCIN>>17  opr=+  inp1=P  carry=CIN  dbl_ovrd=off  block_type=constant
  Constant2 : Constant  Value=0
  Constant3 : xbsIndex_r4/Constant  const=0  gui_display_data_type=Fixed-point  arith_type=Unsigned  n_bits=25  bin_pt=0  preci_type=Single  exp_width=8  frac_width=24  explicit_period=on  period=1  equ=P=C  opselect=C  inp2=PCIN>>17  opr=+  inp1=P  carry=CIN  dbl_ovrd=off  block_type=constant
      settings: block_version=11.4
  Constant4 : xbsIndex_r4/Constant  const=0  gui_display_data_type=Fixed-point  arith_type=Unsigned  n_bits=1  bin_pt=0  preci_type=Single  exp_width=8  frac_width=24  explicit_period=on  period=1  equ=P=C  opselect=C  inp2=PCIN>>17  opr=+  inp1=P  carry=CIN  dbl_ovrd=off  block_type=constant
      settings: block_version=11.4
  Constant5 : xbsIndex_r4/Constant  const=0  gui_display_data_type=Fixed-point  arith_type=Unsigned  n_bits=1  bin_pt=0  preci_type=Single  exp_width=8  frac_width=24  explicit_period=on  period=1  equ=P=C  opselect=C  inp2=PCIN>>17  opr=+  inp1=P  carry=CIN  dbl_ovrd=off  block_type=constant
      settings: block_version=11.4
  Constant6 : xbsIndex_r4/Constant  const=0  gui_display_data_type=Fixed-point  arith_type=Unsigned  n_bits=25  bin_pt=0  preci_type=Single  exp_width=8  frac_width=24  explicit_period=on  period=1  equ=P=C  opselect=C  inp2=PCIN>>17  opr=+  inp1=P  carry=CIN  dbl_ovrd=off  block_type=constant
      settings: block_version=11.4
  Delay{,1..4} (5 alike) : xbsIndex_r4/Delay  rst=off  infoeditControl=Selection of Reset will increase slice count due to use of real FFs and instead of SRLs  en=off  latency=1  dbl_ovrd=off  reg_retiming=off  block_type=delay
  Delay5 : xbsIndex_r4/Delay  rst=off  infoeditControl=Selection of Reset will increase slice count due to use of real FFs and instead of SRLs  en=off  latency=3  dbl_ovrd=off  reg_retiming=off  block_type=delay
  Delay6 : xbsIndex_r4/Delay  rst=off  infoeditControl=Selection of Reset will increase slice count due to use of real FFs and instead of SRLs  en=off  latency=3  dbl_ovrd=off  reg_retiming=off  block_type=delay
  Delay7 : xbsIndex_r4/Delay  rst=off  infoeditControl=Selection of Reset will increase slice count due to use of real FFs and instead of SRLs  en=off  latency=3  dbl_ovrd=off  reg_retiming=off  block_type=delay
  Terminator{1,3..10,13..15} (12 alike) : Terminator
  dest : Subsystem
  gbe_gpu_en : Subsystem
  gbe_sw_en : Subsystem
  gpu : xps_library/ten_Gbe_v2  Tag=xps:tengbe_v2  flavour=sfp+  slot=1  port_r1=0  port_r2_cx4=0  port_r2_sfpp=3  rx_dist_ram=on  large_frames=on  show_param=on  pre_emph_r2=0.74  pre_emph=3  post_emph_r2=0.18  rxeqmix_r2=7  swing_r2=940  swing=800  fab_en=on  fab_mac=hex2dec('0202c0a80501')  fab_ip=hex2dec('c0a80501')  fab_udp=8511  fab_gate=1  cpu_rx_en=off  cpu_tx_en=off
  gpu_mon : Subsystem
  gpu_oflows : xps_library/software register  Tag=xps:sw_reg  io_dir=To Processor  arith_type=Unsigned  bitwidth=32  bin_pt=0  sample_period=1  gw_name=roach2_fengine_orig_eth_3_gpu_oflows_user_data_in
  gpu_status : xps_library/software register  Tag=xps:sw_reg  io_dir=To Processor  arith_type=Unsigned  bitwidth=32  bin_pt=0  sample_period=1  gw_name=roach2_fengine_orig_eth_3_gpu_status_user_data_in
  sw : xps_library/ten_Gbe_v2  Tag=xps:tengbe_v2  flavour=sfp+  slot=1  port_r1=0  port_r2_cx4=0  port_r2_sfpp=2  rx_dist_ram=off  large_frames=on  show_param=on  pre_emph_r2=0.74  pre_emph=3  post_emph_r2=0.18  rxeqmix_r2=7  swing_r2=940  swing=800  fab_en=on  fab_mac=hex2dec('02020a0a0a38')  fab_ip=hex2dec('0a0a0a38')  fab_udp=8511  fab_gate=1  cpu_rx_en=off  cpu_tx_en=off
  sw_bframes : xps_library/software register  Tag=xps:sw_reg  io_dir=To Processor  arith_type=Unsigned  bitwidth=32  bin_pt=0  sample_period=1  gw_name=roach2_fengine_orig_eth_3_sw_bframes_user_data_in
  sw_mon : Subsystem
  sw_oflows : xps_library/software register  Tag=xps:sw_reg  io_dir=To Processor  arith_type=Unsigned  bitwidth=32  bin_pt=0  sample_period=1  gw_name=roach2_fengine_orig_eth_3_sw_oflows_user_data_in
  sw_oruns : xps_library/software register  Tag=xps:sw_reg  io_dir=To Processor  arith_type=Unsigned  bitwidth=32  bin_pt=0  sample_period=1  gw_name=roach2_fengine_orig_eth_3_sw_oruns_user_data_in
  sw_status : xps_library/software register  Tag=xps:sw_reg  io_dir=To Processor  arith_type=Unsigned  bitwidth=32  bin_pt=0  sample_period=1  gw_name=roach2_fengine_orig_eth_3_sw_status_user_data_in
  xip : xps_library/software register  Tag=xps:sw_reg  io_dir=From Processor  arith_type=Unsigned  bitwidth=32  bin_pt=0  sample_period=1  gw_name=roach2_fengine_orig_eth_3_xip_user_data_out
  wires:
  sw_status/1 -> Terminator9/1
  sw_oruns/1 -> Terminator8/1
  sw_oflows/1 -> Terminator7/1
  sw_bframes/1 -> Terminator4/1
  gpu_status/1 -> Terminator3/1
  gpu_oflows/1 -> Terminator1/1
  Bus Selector/1 -> Delay7/1  "<dout>"
  Bus Selector/2 -> Delay6/1  "<valid>"
  data/1 -> Bus Selector3/1, Bus Selector/1, Bus Selector1/1
  Bus Selector1/1 -> Delay5/1  "<eof>"
  Constant/1 -> sw/5
  sw/6 -> Delay2/1
  sw/7 -> sw/7, gbe_gpu_en/1(in)
  sw/10 -> Delay1/1
  dest/1(Out1) -> sw/4
  Constant1/1 -> gpu/5
  sw/12 -> sw/8, [gbe_sw_rx_orun]
  gpu/12 -> gpu/8, [gbe_gpu_rx_orun]
  gpu/7 -> gpu/7
  [gbe_sw_rst] -> sw/1
  [gbe_gpu_rst] -> gpu/1
  gbe_sw_en/1(out) -> sw/3
  gbe_gpu_en/1(out) -> gpu/3
  sw/1 -> [gbe_sw_led_up]
  sw/2 -> [gbe_sw_led_rx]
  sw/3 -> [gbe_sw_led_tx]
  sw/4 -> [gbe_sw_tx_afull]
  sw/5 -> [gbe_sw_tx_oflow]
  sw/8 -> Terminator5/1
  sw/9 -> Terminator6/1
  sw/11 -> [gbe_sw_rx_bfr]
  gpu/1 -> [gbe_gpu_led_up]
  gpu/2 -> [gbe_gpu_led_rx]
  gpu/3 -> [gbe_gpu_led_tx]
  gpu/4 -> [gbe_gpu_tx_afull]
  gpu/5 -> [gbe_gpu_tx_oflow]
  gpu/6 -> Terminator10/1
  gpu/8 -> Terminator14/1
  gpu/9 -> Terminator15/1
  gpu/10 -> Terminator13/1
  gpu/11 -> [gbe_gpu_rx_bfr]
  [gbe_sw_rx_bfr] -> sw_mon/1(bfr)
  [gbe_sw_rx_orun] -> sw_mon/2(orun)
  [gbe_sw_tx_oflow] -> sw_mon/3(oflow)
  Concat/1 -> Delay3/1
  Constant3/1 -> Concat/1
  [gbe_sw_led_up] -> Concat/2
  [gbe_sw_led_rx] -> Concat/3
  [gbe_sw_led_tx] -> Concat/4
  [gbe_sw_tx_afull] -> Concat/5
  [gbe_sw_tx_oflow] -> Concat/6
  [gbe_sw_rx_bfr] -> Concat/7
  [gbe_sw_rx_orun] -> Concat/8
  Concat1/1 -> Delay4/1
  Constant6/1 -> Concat1/1
  [gbe_gpu_led_up] -> Concat1/2
  [gbe_gpu_led_rx] -> Concat1/3
  [gbe_gpu_led_tx] -> Concat1/4
  [gbe_gpu_tx_afull] -> Concat1/5
  [gbe_gpu_tx_oflow] -> Concat1/6
  Constant5/1 -> Concat1/7
  Constant4/1 -> Concat1/8
  Bus Selector3/1 -> dest/1(In1)  "<dest>"
  Delay/1 -> gpu/4
  xip/1 -> Delay/1
  Constant2/1 -> xip/1
  Delay2/1 -> gpu/2
  Delay1/1 -> gpu/6
  Delay3/1 -> sw_status/1
  Delay4/1 -> gpu_status/1
  sw_mon/1(bfr_cnt) -> sw_bframes/1
  sw_mon/3(oflow_cnt) -> sw_oflows/1
  sw_mon/2(orun_cnt) -> sw_oruns/1
  gpu_mon/1(oflow_cnt) -> gpu_oflows/1
  [gbe_gpu_tx_oflow] -> gpu_mon/1(oflow)
  Delay7/1 -> sw/2
  Delay6/1 -> gbe_sw_en/1(in)
  Delay5/1 -> sw/6
